simulink model "example_simulink_LineFollowerDigitalInput"  (Simulink 7.0)
settings: Solver=FixedStepDiscrete  StartTime=0.0  StopTime=inf  FixedStep=20  RelTol=1e-3
libraries: lib_robotinohardware x15
settings Model: Creator=indorewala  LastModifiedBy=ciesla

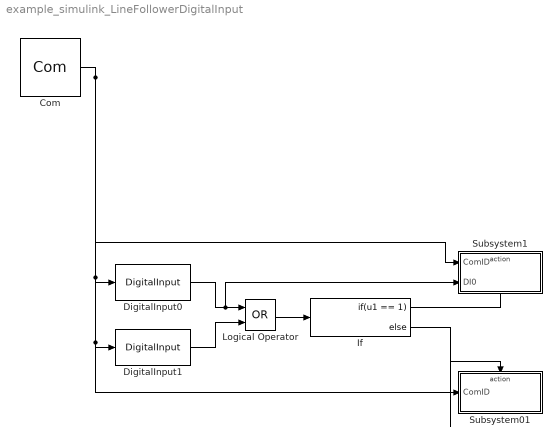
== system example_simulink_LineFollowerDigitalInput ==
  Com : lib_robotinohardware/Com  ip='127.0.0.1'
  DigitalInput0 : lib_robotinohardware/DigitalInput  num=0
  DigitalInput1 : lib_robotinohardware/DigitalInput  num=1
  If : If  IfExpression=u1 == 1
  Logical Operator : Logic  Operator=OR  AllPortsSameDT=off  OutDataTypeMode=boolean
  Subsystem01 : Subsystem  TreatAsAtomicUnit=on
  Subsystem1 : Subsystem  TreatAsAtomicUnit=on
  wires:
  Com/1 -> DigitalInput0/1, DigitalInput1/1, Subsystem01/1(ComID), Subsystem1/1(ComID)
  DigitalInput1/1 -> Logical Operator/2
  DigitalInput0/1 -> Logical Operator/1, Subsystem1/2(DI0)
  If/2 -> Subsystem01/Action
  Logical Operator/1 -> If/1
  If/1 -> Subsystem1/Action

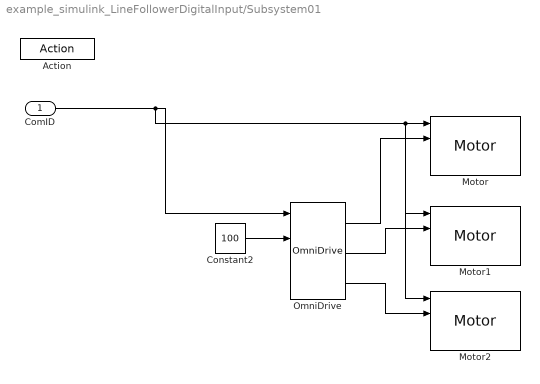
== system example_simulink_LineFollowerDigitalInput/Subsystem01 ==
  ComID : Inport  OutDataType=sfix(16)  OutScaling=2^0
  Action : ActionPort  InitializeStates=reset  ActionType=else
  Constant2 : Constant  Value=100  OutDataType=sfix(16)  OutScaling=2^0
  Motor : lib_robotinohardware/Motor  num=0  kp=255  ki=255  kd=255
  Motor1 : lib_robotinohardware/Motor  num=1  kp=255  ki=255  kd=255
  Motor2 : lib_robotinohardware/Motor  num=2  kp=255  ki=255  kd=255
  OmniDrive : lib_robotinohardware/OmniDrive
  wires:
  Constant2/1 -> OmniDrive/2
  OmniDrive/1 -> Motor/2
  OmniDrive/2 -> Motor1/2
  OmniDrive/3 -> Motor2/2
  ComID/1 -> OmniDrive/1, Motor/1, Motor1/1, Motor2/1

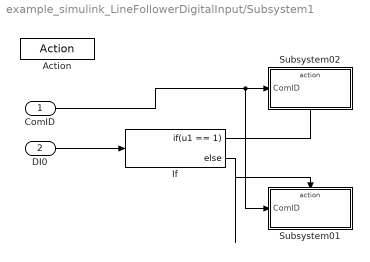
== system example_simulink_LineFollowerDigitalInput/Subsystem1 ==
  ComID : Inport  OutDataType=sfix(16)  OutScaling=2^0
  DI0 : Inport  Port=2  OutDataType=sfix(16)  OutScaling=2^0
  Action : ActionPort  InitializeStates=reset  ActionType=then
  If : If  IfExpression=u1 == 1
  Subsystem01 : Subsystem  TreatAsAtomicUnit=on
  Subsystem02 : Subsystem  TreatAsAtomicUnit=on
  wires:
  DI0/1 -> If/1
  ComID/1 -> Subsystem02/1(ComID), Subsystem01/1(ComID)
  If/1 -> Subsystem02/Action
  If/2 -> Subsystem01/Action

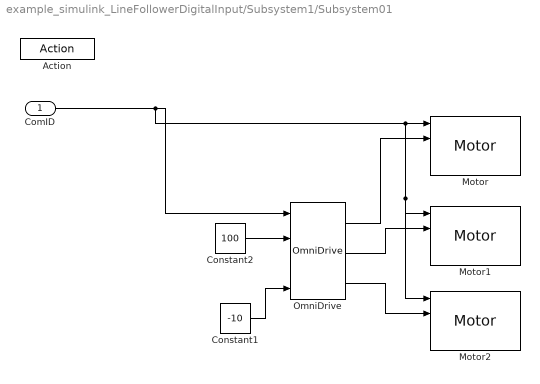
== system example_simulink_LineFollowerDigitalInput/Subsystem1/Subsystem01 ==
  ComID : Inport  OutDataType=sfix(16)  OutScaling=2^0
  Action : ActionPort  InitializeStates=reset  ActionType=else
  Constant1 : Constant  Value=-10  OutDataType=sfix(16)  OutScaling=2^0
  Constant2 : Constant  Value=100  OutDataType=sfix(16)  OutScaling=2^0
  Motor : lib_robotinohardware/Motor  num=0  kp=255  ki=255  kd=255
  Motor1 : lib_robotinohardware/Motor  num=1  kp=255  ki=255  kd=255
  Motor2 : lib_robotinohardware/Motor  num=2  kp=255  ki=255  kd=255
  OmniDrive : lib_robotinohardware/OmniDrive
  wires:
  Constant2/1 -> OmniDrive/2
  OmniDrive/1 -> Motor/2
  OmniDrive/2 -> Motor1/2
  OmniDrive/3 -> Motor2/2
  ComID/1 -> OmniDrive/1, Motor/1, Motor1/1, Motor2/1
  Constant1/1 -> OmniDrive/4

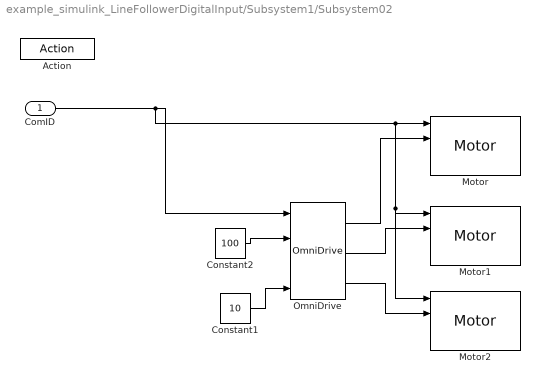
== system example_simulink_LineFollowerDigitalInput/Subsystem1/Subsystem02 ==
  ComID : Inport  OutDataType=sfix(16)  OutScaling=2^0
  Action : ActionPort  InitializeStates=reset  ActionType=then
  Constant1 : Constant  Value=10  OutDataType=sfix(16)  OutScaling=2^0
  Constant2 : Constant  Value=100  OutDataType=sfix(16)  OutScaling=2^0
  Motor : lib_robotinohardware/Motor  num=0  kp=255  ki=255  kd=255
  Motor1 : lib_robotinohardware/Motor  num=1  kp=255  ki=255  kd=255
  Motor2 : lib_robotinohardware/Motor  num=2  kp=255  ki=255  kd=255
  OmniDrive : lib_robotinohardware/OmniDrive
  wires:
  Constant2/1 -> OmniDrive/2
  OmniDrive/1 -> Motor/2
  OmniDrive/2 -> Motor1/2
  OmniDrive/3 -> Motor2/2
  ComID/1 -> OmniDrive/1, Motor/1, Motor1/1, Motor2/1
  Constant1/1 -> OmniDrive/4
